simulink model "PIcontoller"  (R2020b)
settings: Solver=VariableStepAuto  StartTime=0.0  StopTime=10.0  RelTol=1e-3
model workspace (MAT data in the model file):
  K = Simulink.Parameter
  K.Value = 0.0274
  K.DataType = 'auto'
  K.Dimensions = [1 1]
settings Model: Creator=lalit  LastModifiedBy=lalit
settings DataIOCC: SaveOutput=off  SaveTime=off

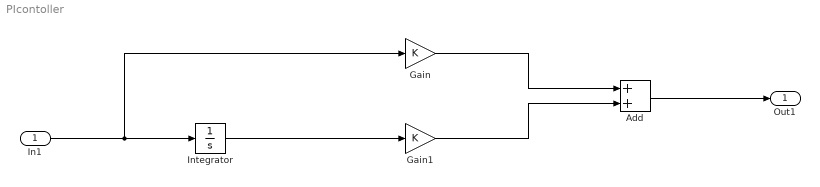
== system PIcontoller ==
  In1 : Inport  OutDataTypeStr=double  PortDimensions=1  SampleTime=0
  Add : Sum
  Gain : Gain  Gain=K
  Gain1 : Gain  Gain=K
  Integrator : Integrator
  Out1 : Outport  OutDataTypeStr=double  PortDimensions=1  SampleTime=0
  wires:
  Gain/1 -> Add/1
  In1/1 -> Integrator/1, Gain/1
  Integrator/1 -> Gain1/1
  Gain1/1 -> Add/2
  Add/1 -> Out1/1
